simulink model "closed_loop_sin"  (R2017a)
settings: Solver=ode4  StartTime=0.0  StopTime=60  FixedStep=0.001  RelTol=1e-3  EnableMultiTasking=on
undefined symbols (not defined in the file): National_Instruments, PCI
libraries: sldrtlib x2
settings Model: SimulationMode=external  ExtModeTrigDuration=300000  ExtModeTrigDurationFloating=300  ExtModeArchiveFileName=Arm motion with Impulse  ExtModeArchiveDirName=E:\work\test1\NachumEisen\Exp1  Creator=test1  LastModifiedBy=me-int1
settings DataIOCC: SaveFormat=Array
settings DebuggingCC: SFUnexpectedBacktrackingDiag=warning  SFNoUnconditionalDefaultTransitionDiag=warning  SFExecutionAtInitializationDiag=none
settings HardwareCC: TargetBitPerLong=64  TargetBitPerPointer=64  TargetIntDivRoundTo=Zero  TargetEndianess=LittleEndian  TargetWordSize=64  TargetHWDeviceType=Intel->x86-64
settings ModelReferenceCC: PropagateSignalLabelsOutOfModel=off
settings RTWCC: SystemTargetFile=sldrt.tlc  TemplateMakefile=sldrt.tmf  Description=Simulink Desktop Real-Time  RTWCompilerOptimization=on
settings CodeAppCC: MaxIdLength=95
settings SimulinkDesktopRealTimeCC: TargetPreCompLibLocation=C:\Program Files\MATLAB\R2017a\toolbox\sldrt\lib\win64  TargetLangStandard=C89/C90 (ANSI)  SupportVariableSizeSignals=off
settings ConfigComp: CovMetricSettings=dw  CovHtmlReporting=on  CovSaveCumulativeToWorkspaceVar=on  CovSaveSingleToWorkspaceVar=on  CovExternalEMLEnable=off

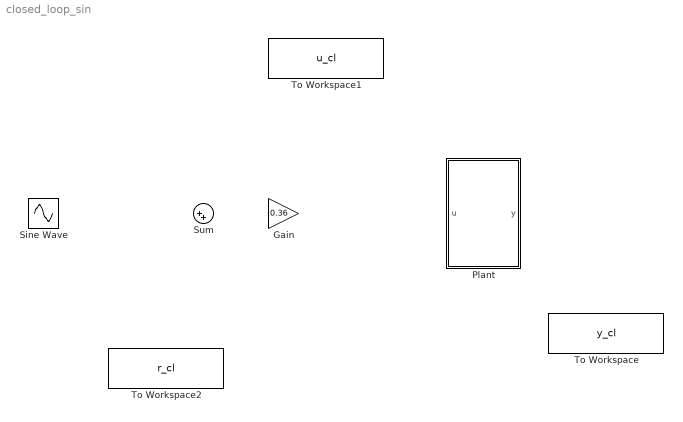
== system closed_loop_sin ==
  Gain : Gain  Gain=0.36
  Plant : Subsystem
  Sine Wave : Sin  Amplitude=10  Frequency=0  SampleTime=0
  Sum : Sum  Inputs=|++
  To Workspace : ToWorkspace  VariableName=y_cl  SaveFormat=Structure With Time  SampleTime=-1
  To Workspace1 : ToWorkspace  VariableName=u_cl  SaveFormat=Structure With Time  SampleTime=-1
  To Workspace2 : ToWorkspace  VariableName=r_cl  SaveFormat=Structure With Time  SampleTime=-1

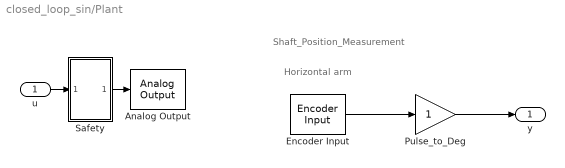
== system closed_loop_sin/Plant ==
  note: Shaft_Position_Measurement
  note: Horizontal arm
  u : Inport
  Analog Output : sldrtlib/Analog Output  SampleTime=0.001  MaxMissedTicks=10  ShowMissedTicks=off  YieldWhenWaiting=off  DrvName=National_Instruments/PCI-6221  DrvAddress=4294967295  DrvOptions=[0 0 0 2 2]  Channels=[2]  RangeMode=1  VoltRange=1  InitialValue=0  FinalValue=0
      settings: AttributesFormatString=National Instruments\nPCI-6221 [auto]  SourceProductName=Simulink Desktop Real-Time
  Encoder Input : sldrtlib/Encoder Input  SampleTime=0.001  MaxMissedTicks=10  ShowMissedTicks=off  YieldWhenWaiting=off  DrvName=National_Instruments/PCI-6221  DrvAddress=4294967295  DrvOptions=[0 0 0 2 2]  Channels=[1]  QuadMode=3  IndexPulse=1  InputFilter=Inf  DataType=1
      settings: AttributesFormatString=National Instruments\nPCI-6221 [auto]  SourceProductName=Simulink Desktop Real-Time
  Pulse_to_Deg : Gain
  Safety : Subsystem
  y : Outport
  wires:
  Pulse_to_Deg/1 -> y/1
  Encoder Input/1 -> Pulse_to_Deg/1
  u/1 -> Safety/1(In1)
  Safety/1(Out1) -> Analog Output/1

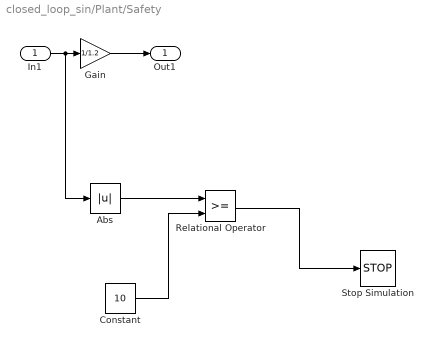
== system closed_loop_sin/Plant/Safety ==
  In1 : Inport
  Abs : Abs
  Constant : Constant  Value=10
  Gain : Gain  Gain=1/1.2
  Relational Operator : RelationalOperator  OutDataTypeStr=boolean  RndMeth=Nearest
  Stop Simulation : Stop
  Out1 : Outport
  wires:
  In1/1 -> Abs/1, Gain/1
  Gain/1 -> Out1/1
  Relational Operator/1 -> Stop Simulation/1
  Constant/1 -> Relational Operator/2
  Abs/1 -> Relational Operator/1
